simulink model "SMC_comparativa"  (R2022b)
settings: Solver=VariableStepAuto  StartTime=0.0  StopTime=10.0  MaxStep=0.02  RelTol=1e-4
undefined symbols (not defined in the file): a, B, beta, d, delta_x1, g, Go, J, Ke, Kt, lambda1, lambda2, m, x10, x20
settings Model: Creator=amoralesma  LastModifiedBy=amoralesma

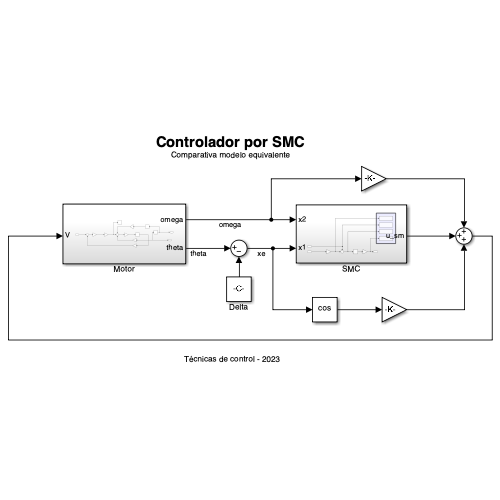
[thumbnail: Simulink's stored preview of the top-level diagram]
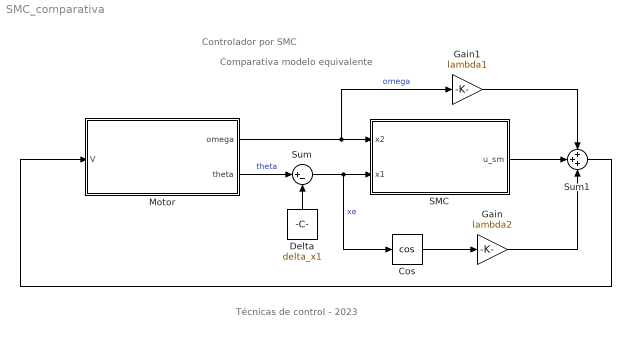
== system SMC_comparativa ==
  note: Técnicas de control - 2023
  note: Comparativa modelo equivalente
  note: Controlador por SMC
  Cos : Trigonometry  Operator=cos
  Delta : Constant  Value=delta_x1
  Gain : Gain  Gain=lambda2
  Gain1 : Gain  Gain=lambda1
  Motor : Subsystem
  SMC : Subsystem
  Sum : Sum  Inputs=|+-
  Sum1 : Sum  Inputs=+++
  wires:
  Motor/1(omega) -> SMC/1(x2), Gain1/1  "omega"
  Motor/2(theta) -> Sum/1  "theta"
  Delta/1 -> Sum/2
  Sum/1 -> Cos/1, SMC/2(x1)  "xe"
  SMC/1(u_sm) -> Sum1/2
  Sum1/1 -> Motor/1(V)
  Gain1/1 -> Sum1/1
  Cos/1 -> Gain/1
  Gain/1 -> Sum1/3

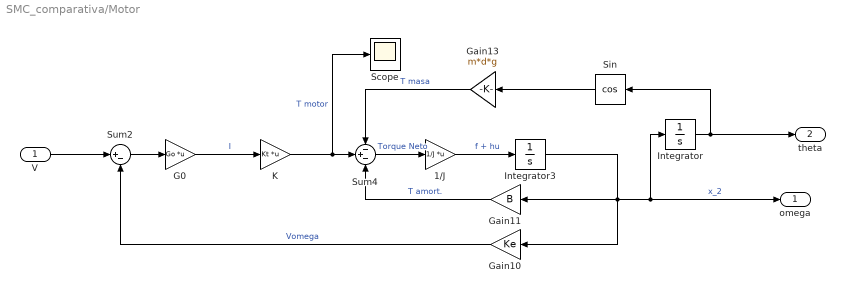
== system SMC_comparativa/Motor ==
  V : Inport
  1/J : Gain  Gain=1/J  Multiplication=Matrix(K*u)
  G0 : Gain  Gain=Go  Multiplication=Matrix(K*u)
  Gain10 : Gain  Gain=Ke
  Gain11 : Gain  Gain=B
  Gain13 : Gain  Gain=m*d*g
  Integrator : Integrator  InitialCondition=x10  ZeroCross=off
  Integrator3 : Integrator  InitialCondition=x20  ZeroCross=off
  K : Gain  Gain=Kt  Multiplication=Matrix(K*u)
  Scope : Scope
  Sin : Trigonometry  Operator=cos
  Sum2 : Sum  Inputs=|+-
  Sum4 : Sum  Inputs=-+-
  omega : Outport
  theta : Outport  Port=2
  wires:
  Gain10/1 -> Sum2/2  "Vomega"
  Sum4/1 -> 1/J/1  "Torque Neto"
  Integrator3/1 -> Gain11/1, Gain10/1, Integrator/1, omega/1  "x_2"
  Gain11/1 -> Sum4/3  "T amort."
  Sum2/1 -> G0/1
  K/1 -> Scope/1, Sum4/2  "T motor"
  1/J/1 -> Integrator3/1  "f + hu"
  G0/1 -> K/1  "I"
  V/1 -> Sum2/1
  Integrator/1 -> Sin/1, theta/1
  Sin/1 -> Gain13/1
  Gain13/1 -> Sum4/1  "T masa"

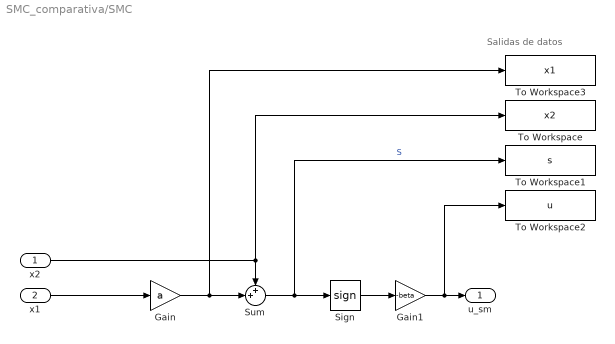
== system SMC_comparativa/SMC ==
  note: Salidas de datos
  x2 : Inport
  x1 : Inport  Port=2
  Gain : Gain  Gain=a
  Gain1 : Gain  Gain=-beta
  Sign : Signum  ZeroCross=off
  Sum : Sum  Inputs=++|
  To Workspace : ToWorkspace  VariableName=x2  SaveFormat=Timeseries  SampleTime=-1
  To Workspace1 : ToWorkspace  VariableName=s  SaveFormat=Timeseries  SampleTime=-1
  To Workspace2 : ToWorkspace  VariableName=u  SaveFormat=Timeseries  SampleTime=-1
  To Workspace3 : ToWorkspace  VariableName=x1  SaveFormat=Timeseries  SampleTime=-1
  u_sm : Outport
  wires:
  x1/1 -> Gain/1
  Sum/1 -> Sign/1, To Workspace1/1  "S"
  x2/1 -> To Workspace/1, Sum/1
  Gain/1 -> To Workspace3/1, Sum/2
  Sign/1 -> Gain1/1
  Gain1/1 -> To Workspace2/1, u_sm/1
